simulink model "PID"  (R2021b)
settings: Solver=FixedStepDiscrete  StartTime=0.0  StopTime=10.0  FixedStep=0.01  RelTol=1e-3
undefined symbols (not defined in the file): Kd_Pt, Ki_Pt, Kp_Pt, Ts_Cn
settings Model: Creator=banashreen  LastModifiedBy=Dell-pc
settings SolverCC: AlgebraicLoopSolver=TrustRegion
settings DataIOCC: ReturnWorkspaceOutputs=off
settings OptimizationCC: DefaultParameterBehavior=Inlined  PassReuseOutputArgsAs=Individual arguments  EfficientTunableParamExpr=on
settings DebuggingCC: ParameterTunabilityLossMsg=error  SFMachineParentedDataDiag=warning  ArithmeticOperatorsInVariantConditions=warning
settings SFSimCC: SimUseLocalCustomCode=off  MATLABDynamicMemAlloc=off  CustomCodeUndefinedFunction=UseInterfaceOnly
settings RTWCC: Description=Embedded Coder  SystemTargetFile=ert.tlc  TemplateMakefile=ert_default_tmf  GenerateReport=on  RTWUseLocalCustomCode=off  IncludeHyperlinkInReport=on  LaunchReport=on  GenerateTraceInfo=on  GenerateTraceReport=on  GenerateTraceReportSl=on  GenerateTraceReportSf=on  GenerateTraceReportEml=on
settings CodeAppCC: ForceParamTrailComments=on  IgnoreCustomStorageClasses=off  OperatorAnnotations=on  SimulinkDataObjDesc=on  SFDataObjDesc=on  InsertBlockDesc=on
settings ERTTargetCC: TargetLangStandard=C99 (ISO)  GenerateSampleERTMain=on  InlinedParameterPlacement=NonHierarchical  ERTCustomFileTemplate=example_file_process.tlc

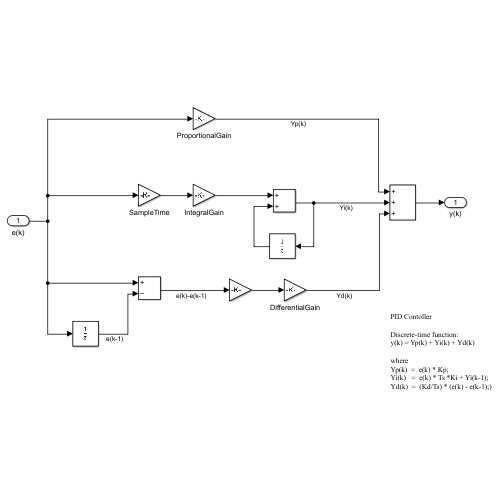
[thumbnail: Simulink's stored preview of the top-level diagram]
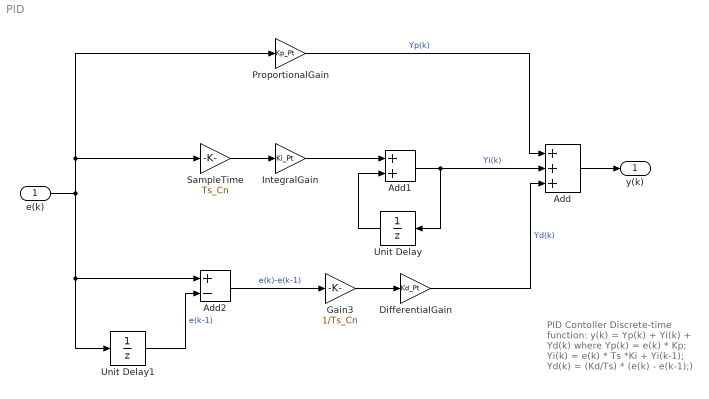
== system PID ==
  note: PID Contoller
      |
      | Discrete-time function:
      | y(k) = Yp(k) + Yi(k) + Yd(k)
      |
      | where
      | Yp(k) = e(k) * Kp;
      | Yi(k) = e(k) * Ts *Ki + Yi(k-1);
      | Yd(k) = (Kd/Ts) * (e(k) - e(k-1);)
  e(k) : Inport
  Add : Sum  Inputs=+++
  Add1 : Sum
  Add2 : Sum  Inputs=+-  AccumDataTypeStr=single
  DifferentialGain : Gain  Gain=Kd_Pt  OutDataTypeStr=single
  Gain3 : Gain  Gain=1/Ts_Cn  OutDataTypeStr=single
  IntegralGain : Gain  Gain=Ki_Pt
  ProportionalGain : Gain  Gain=Kp_Pt  OutDataTypeStr=single
  SampleTime : Gain  Gain=Ts_Cn  OutDataTypeStr=single
  Unit Delay : UnitDelay  SampleTime=-1  HasFrameUpgradeWarning=on
  Unit Delay1 : UnitDelay  SampleTime=-1  HasFrameUpgradeWarning=on
  y(k) : Outport  VectorParamsAs1DForOutWhenUnconnected=off
  wires:
  ProportionalGain/1 -> Add/1  "Yp(k)"
  SampleTime/1 -> IntegralGain/1
  IntegralGain/1 -> Add1/1
  Add1/1 -> Add/2, Unit Delay/1  "Yi(k)"
  Unit Delay/1 -> Add1/2
  Unit Delay1/1 -> Add2/2  "e(k-1)"
  Add2/1 -> Gain3/1  "e(k)-e(k-1)"
  Gain3/1 -> DifferentialGain/1
  DifferentialGain/1 -> Add/3  "Yd(k)"
  Add/1 -> y(k)/1
  e(k)/1 -> SampleTime/1, ProportionalGain/1, Add2/1, Unit Delay1/1
